simulink model "W01_rc_usb"  (R2024b)
settings: Solver=ode4  StartTime=0  StopTime=inf  FixedStep=h  RelTol=1e-3
PostLoadFcn:
  | p_ = fileparts(get_param(bdroot,'FileName')); addpath(p_, fullfile(fileparts(fileparts(p_)),'_tools')); mss_path(); clear p_
StartFcn:
  | if isappdata(0,'W01rc_tap'), rmappdata(0,'W01rc_tap'); end; setappdata(0,'W01rc_model',bdroot);
model workspace (MAT data in the model file):
  Binv = [0.5  1.26582278481; 0.5  -1.26582278481]
  Bxn = [1  1; 0.395  -0.395]
  N_max = 52.69932
  V_c = 0
  X_max = 239.364
  Xu_abs = 77.5544323484
  animate = 1
  beta_c = 0
  h = 0.02
  js_rud = 4
  js_sgn = [1 1]
  js_thr = 3
  k_neg = 0.006445
  k_pos = 0.01108
  mp = 25
  n_max = 103.930864274
  n_min = -101.736665504
  rp = [0.05; 0; -0.35]
  x0 = [0; 0; 0; 0; 0; 0; 0; 0; 0; 0; 0; 0]
libraries: vrlib x1
settings Model: Creator=admin  LastModifiedBy=admin
settings DataIOCC: ReturnWorkspaceOutputs=off
settings OptimizationCC: BlockReduction=off

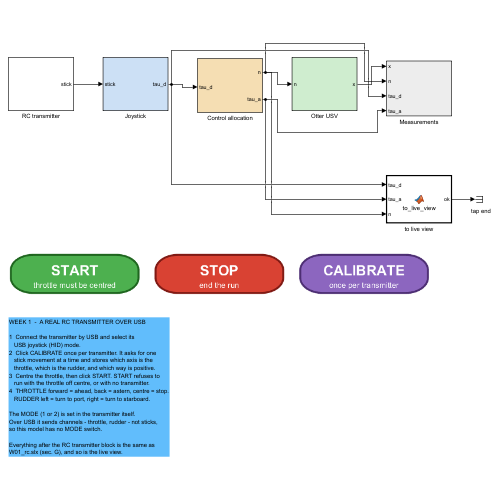
[thumbnail: Simulink's stored preview of the top-level diagram]
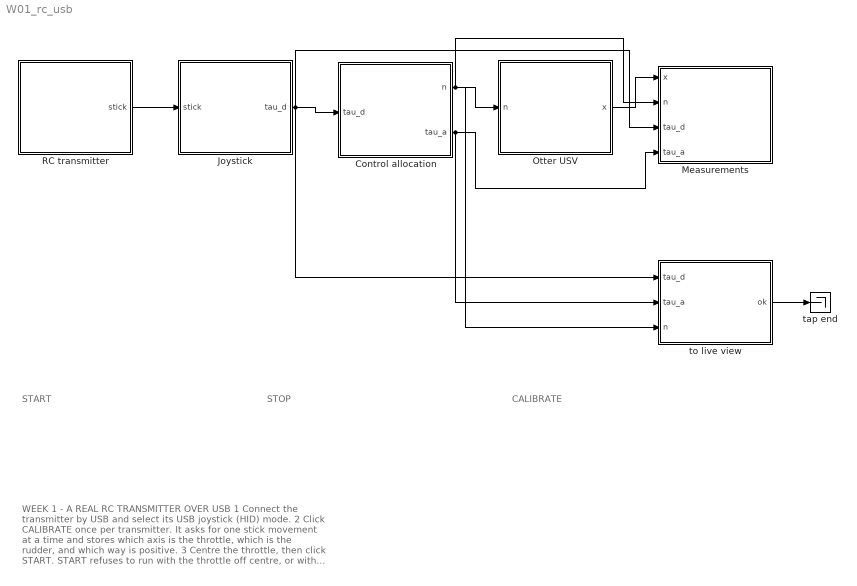
== system W01_rc_usb ==
  note: START
  note: STOP
  note: CALIBRATE
  note: WEEK 1  -  A REAL RC TRANSMITTER OVER USB
      |
      | 1  Connect the transmitter by USB and select its
      |    USB joystick (HID) mode.
      | 2  Click CALIBRATE once per transmitter. It asks for one
      |    stick movement at a time and stores which axis is the
      |    throttle, which is the rudder, and which way is positive.
      | 3  Centre the throttle, then click START. START refuses to
      |    run with the throttle off centre, or with no transmitter.
      | 4  THROTTLE forward = ahead, back = astern, centre = stop.
      |    RUDDER left = turn to port, right = turn to starboard.
      |
      | The MODE (1 or 2) is set in the transmitter itself.
      | Over USB it sends channels - throttle, rudder - not sticks,
      | so this model has no MODE switch.
      |
      | Everything after the RC transmitter block is the same as
      | W01_rc.slx (sec. G), and so is the live view.
  Control allocation : Subsystem
  Joystick : Subsystem
  Measurements : Subsystem
  Otter USV : Subsystem
  RC transmitter : Subsystem
  tap end : Terminator
  to live view : MATLAB Function  TreatAsAtomicUnit=on
  wires:
  RC transmitter/1(stick) -> Joystick/1(stick)
  Joystick/1(tau_d) -> Control allocation/1(tau_d), Measurements/3(tau_d), to live view/1(tau_d)
  Control allocation/1(n) -> Otter USV/1(n), Measurements/2(n), to live view/3(n)
  Otter USV/1(x) -> Measurements/1(x)
  Control allocation/2(tau_a) -> Measurements/4(tau_a), to live view/2(tau_a)
  to live view/1(ok) -> tap end/1

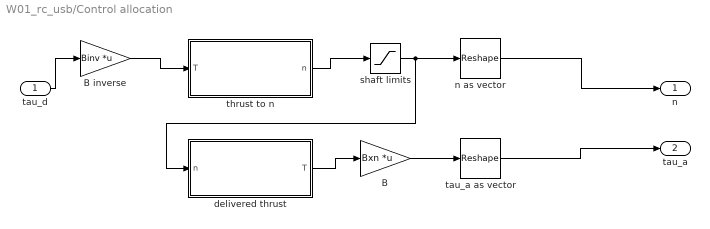
== system W01_rc_usb/Control allocation ==
  tau_d : Inport
  B : Gain  Gain=Bxn  Multiplication=Matrix(K*u)
  B inverse : Gain  Gain=Binv  Multiplication=Matrix(K*u)
  delivered thrust : MATLAB Function  TreatAsAtomicUnit=on
  n as vector : Reshape
  shaft limits : Saturate  UpperLimit=n_max  LowerLimit=n_min
  tau_a as vector : Reshape
  thrust to n : MATLAB Function  TreatAsAtomicUnit=on
  n : Outport
  tau_a : Outport  Port=2
  wires:
  tau_d/1 -> B inverse/1
  B inverse/1 -> thrust to n/1(T)
  thrust to n/1(n) -> shaft limits/1
  shaft limits/1 -> n as vector/1, delivered thrust/1(n)
  n as vector/1 -> n/1
  delivered thrust/1(T) -> B/1
  B/1 -> tau_a as vector/1
  tau_a as vector/1 -> tau_a/1

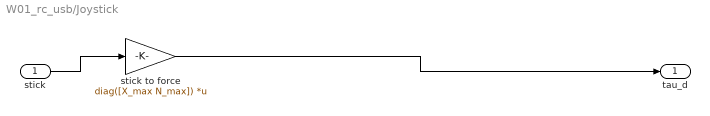
== system W01_rc_usb/Joystick ==
  stick : Inport
  stick to force : Gain  Gain=diag([X_max N_max])  Multiplication=Matrix(K*u)
  tau_d : Outport
  wires:
  stick/1 -> stick to force/1
  stick to force/1 -> tau_d/1

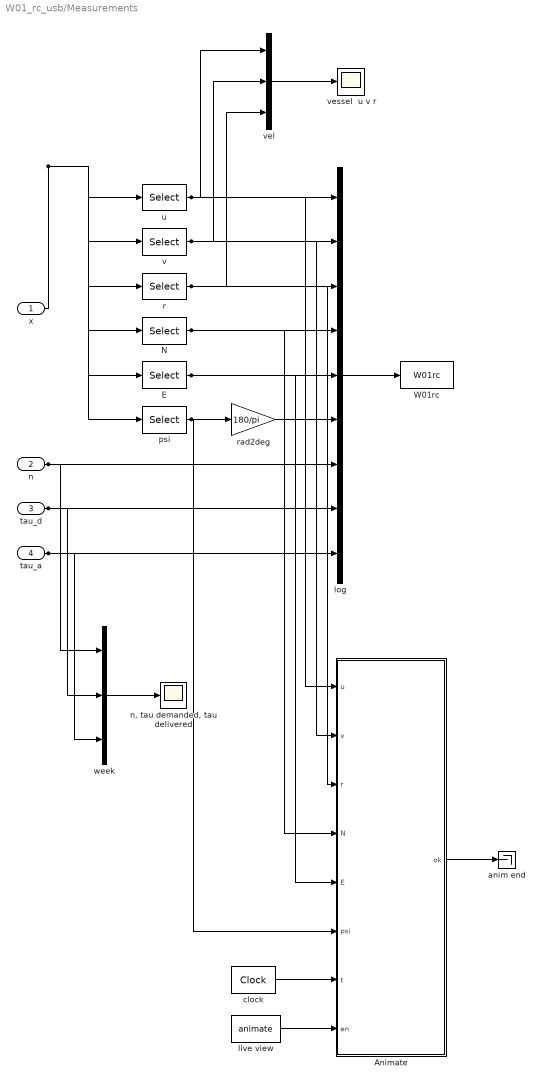
== system W01_rc_usb/Measurements ==
  x : Inport
  n : Inport  Port=2
  tau_d : Inport  Port=3
  tau_a : Inport  Port=4
  Animate : MATLAB Function  TreatAsAtomicUnit=on
  E : Selector  InputPortWidth=12  IndexOptions=Index vector (dialog)  Indices=8  OutputSizes=1
  N : Selector  InputPortWidth=12  IndexOptions=Index vector (dialog)  Indices=7  OutputSizes=1
  W01rc : ToWorkspace  VariableName=W01rc  SaveFormat=Structure With Time  SampleTime=-1
  anim end : Terminator
  clock : DigitalClock  SampleTime=h
  live view : Constant  Value=animate
  log : Mux  Inputs=9
  "n, tau demanded, tau delivered" : Scope
  psi : Selector  InputPortWidth=12  IndexOptions=Index vector (dialog)  Indices=12  OutputSizes=1
  r : Selector  InputPortWidth=12  IndexOptions=Index vector (dialog)  Indices=6  OutputSizes=1
  rad2deg : Gain  Gain=180/pi
  u : Selector  InputPortWidth=12  IndexOptions=Index vector (dialog)  Indices=1  OutputSizes=1
  v : Selector  InputPortWidth=12  IndexOptions=Index vector (dialog)  Indices=2  OutputSizes=1
  vel : Mux  Inputs=3
  vessel  u v r : Scope
  week : Mux  Inputs=3
  wires:
  x/1 -> u/1, v/1, r/1, N/1, E/1, psi/1
  log/1 -> W01rc/1
  psi/1 -> rad2deg/1, Animate/6(psi)
  u/1 -> log/1, vel/1, Animate/1(u)
  v/1 -> log/2, vel/2, Animate/2(v)
  r/1 -> log/3, vel/3, Animate/3(r)
  N/1 -> log/4, Animate/4(N)
  E/1 -> log/5, Animate/5(E)
  rad2deg/1 -> log/6
  n/1 -> log/7, week/1
  tau_d/1 -> log/8, week/2
  tau_a/1 -> log/9, week/3
  vel/1 -> vessel  u v r/1
  week/1 -> "n, tau demanded, tau delivered"/1
  clock/1 -> Animate/7(t)
  live view/1 -> Animate/8(en)
  Animate/1(ok) -> anim end/1

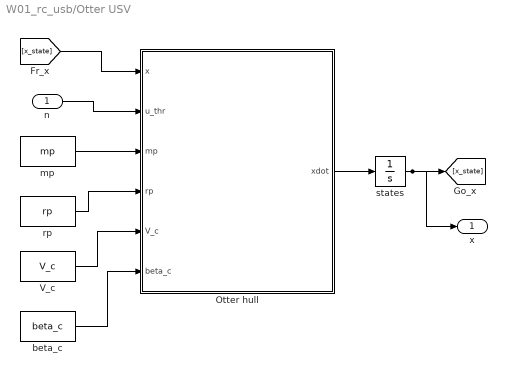
== system W01_rc_usb/Otter USV ==
  n : Inport
  Otter hull : MATLAB Function  TreatAsAtomicUnit=on
  V_c : Constant  Value=V_c
  beta_c : Constant  Value=beta_c
  mp : Constant  Value=mp
  rp : Constant  Value=rp
  states : Integrator  InitialCondition=x0
  x : Outport
  wires:
  states/1 -> [x_state], x/1
  [x_state] -> Otter hull/1(x)
  V_c/1 -> Otter hull/5(V_c)
  mp/1 -> Otter hull/3(mp)
  n/1 -> Otter hull/2(u_thr)
  Otter hull/1(xdot) -> states/1
  beta_c/1 -> Otter hull/6(beta_c)
  rp/1 -> Otter hull/4(rp)

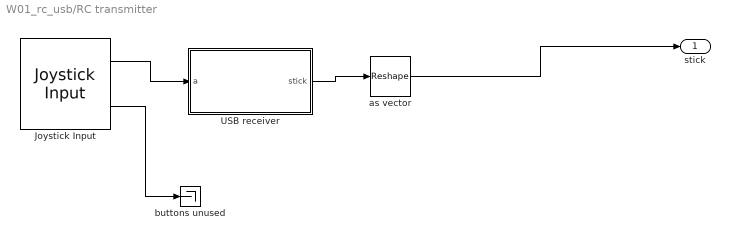
== system W01_rc_usb/RC transmitter ==
  Joystick Input : vrlib/Joystick Input  joyid=1  adjustports=on  forcefeed=off
  USB receiver : MATLAB Function  TreatAsAtomicUnit=on
  as vector : Reshape
  buttons unused : Terminator
  stick : Outport
  wires:
  Joystick Input/1 -> USB receiver/1(a)
  USB receiver/1(stick) -> as vector/1
  as vector/1 -> stick/1
  Joystick Input/2 -> buttons unused/1

== matlab function W01_rc_usb/Control allocation/thrust to n ==
  data: T input; n output double size=[2 1]; k_pos parameter; k_neg parameter
function n = thrust_to_n(T, k_pos, k_neg)
%#codegen
%THRUST_TO_N  Invert the propeller curve of sec. 1-10, one propeller at a time.
%
%   T = k n|n| with k = k_pos ahead and k_neg astern, so
%   n = sign(T) sqrt(|T| / k). The coefficient is chosen by the sign of the
%   demanded thrust, which is also the sign of the shaft speed.
n = zeros(2,1);
for i = 1:2
    if T(i) >= 0
        n(i) =  sqrt( T(i) / k_pos);
    else
        n(i) = -sqrt(-T(i) / k_neg);
    end
end

== matlab function W01_rc_usb/RC transmitter/USB receiver ==
  data: a input; stick output double size=[2 1]; js_thr parameter; js_rud parameter; js_sgn parameter
function stick = usb_receiver(a, js_thr, js_rud, js_sgn)
%#codegen
%USB_RECEIVER  Two axes of a USB transmitter to [s_T; s_R], each -1..+1.
%
%   A transmitter in USB joystick mode sends its CHANNELS, not its sticks:
%   the mode (1 or 2) is applied inside the transmitter, so the throttle is
%   the same axis whichever hand moves it. js_thr and js_rud say which axis
%   is which, js_sgn which way is positive. W01_H_usb_setup finds all three.
%
%   Each axis, -1..+1, is turned into the 0..100 channel of the on-screen
%   model and passed through the same neutral zone, so the two models give
%   the same stick deflection for the same stick position.
db = 3;                                   % neutral zone [% of travel]
stick = zeros(2,1);
k = [js_thr; js_rud];
for i = 1:2
    if k(i) >= 1 && k(i) <= numel(a)
        d = 50 * js_sgn(i) * double(a(k(i)));
        stick(i) = sign(d) * max(abs(d) - db, 0) / (50 - db);
    end
end
stick = min(max(stick, -1), 1);

== matlab function W01_rc_usb/Control allocation/delivered thrust ==
  data: n input; T output double size=[2 1]; k_pos parameter; k_neg parameter
function T = delivered_thrust(n, k_pos, k_neg)
%#codegen
%DELIVERED_THRUST  The thrust the propellers give at the saturated speed.
%
%   The same curve as otter.m lines 165-177. Below saturation this returns
%   the demanded thrust exactly; at saturation it returns less, and the
%   difference is what the operator asked for and did not get.
T = zeros(2,1);
for i = 1:2
    if n(i) > 0
        T(i) = k_pos * n(i) * abs(n(i));
    else
        T(i) = k_neg * n(i) * abs(n(i));
    end
end

== matlab function W01_rc_usb/Otter USV/Otter hull ==
  data: x input; xdot output double size=[12 1]; u_thr input; mp input; rp input; V_c input; beta_c input
function xdot = otter_hull(x, u_thr, mp, rp, V_c, beta_c)
% Fossen's otter.m, called unchanged from Tools/MSS/VESSELS.
%
%   x       12 states, fed back from the integrator
%   u_thr   propeller shaft speeds [rad/s]
%
% otter.m is not written for code generation, so the call is extrinsic and
% xdot has to be pre-sized for Simulink to know the output width.
coder.extrinsic('otter');

xdot = zeros(12,1);
xdot = otter(x, u_thr, mp, rp, V_c, beta_c);
end

== matlab function W01_rc_usb/Measurements/Animate ==
  data: u input; ok output; v input; r input; N input; E input; psi input; t input; en input
function ok = Animate(u, v, r, N, E, psi, t, en)
%#codegen
% Live view of the vessel while the model runs.
%
% A MATLAB Function block cannot plot, so the drawing function is declared
% extrinsic: Simulink calls plain MATLAB rather than generating code for it.
% Set animate = 0 in the setup script to switch the live view off.
%
% psi arrives in RADIANS and r in rad/s - the units otter.m works in. The
% wrapper converts them for display, in one place, so no two figures in the
% course can disagree about what a degree is.
coder.extrinsic('W01rc_animate');
ok = 1;
if en > 0.5
    W01rc_animate(u, v, r, N, E, psi, t);
end
end

== matlab function W01_rc_usb/to live view ==
  data: tau_d input; ok output double size=1; tau_a input; n input
function ok = to_live_view(tau_d, tau_a, n)
%#codegen
%TO_LIVE_VIEW  Hand the demand, the delivery and the shaft speeds to the live view.
%
%   The Animate block inside Measurements receives only the vessel states.
%   W01rc_animate reads these six numbers from here at every step.
coder.extrinsic('setappdata');
setappdata(0, 'W01rc_tap', [tau_d(:); tau_a(:); n(:)]);
ok = 1;
